simulink model "LinStSpace_org"  (Simulink 10.0)
settings: Solver=ode3  StartTime=0.0  StopTime=20  FixedStep=1  RelTol=1e-3  EnableMultiTasking=on
libraries: Lib_Solve_Linearize_TMATS x1
settings Model: Creator=jwchapm2  LastModifiedBy=annonymous
settings DataIOCC: LimitDataPoints=on  SignalLoggingSaveFormat=ModelDataLogs
settings DebuggingCC: UnderspecifiedInitializationDetection=Simplified  MergeDetectMultiDrivingBlocksExec=error  SolverPrmCheckMsg=warning  MultiTaskDSMMsg=warning  MultiTaskCondExecSysMsg=none  StrictBusMsg=WarnOnBusTreatedAsVector  NonBusSignalsTreatedAsBus=warning
settings GRTTargetCC: GeneratePreprocessorConditionals=Disable all  CombineOutputUpdateFcns=on  GRTInterface=off
settings ConfigComp: CovExternalEMLEnable=off

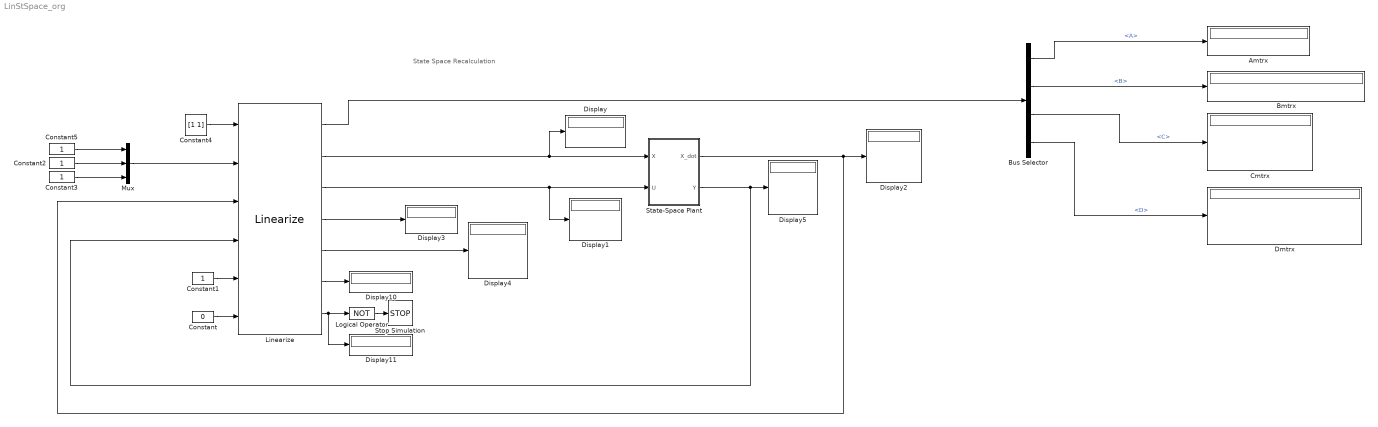
== system LinStSpace_org ==
  note: State Space Recalculation
  Amtrx : Display
  Bmtrx : Display
  Bus Selector : BusSelector  OutputSignals=A,B,C,D
  Cmtrx : Display
  Constant : Constant  Value=0
  Constant{1..3,5} (4 alike) : Constant
  Constant4 : Constant  Value=[1 1]
  Display{,1..5,10..11} (8 alike) : Display
  Dmtrx : Display
  Linearize : Lib_Solve_Linearize_TMATS/Linearize  N_XPer_M=[0.01 0.01;-0.01 -0.01]  N_UPer_M=[0.01 0.01 0.01;-0.01 -0.01 -0.01]  N_Y_M=4
  Logical Operator : Logic  Operator=NOT  AllPortsSameDT=off  OutDataTypeStr=boolean
  Mux : Mux  Inputs=3
  State-Space Plant : Subsystem
  Stop Simulation : Stop
  wires:
  Linearize/2 -> Display/1, State-Space Plant/1(X)
  Linearize/1 -> Bus Selector/1
  Linearize/4 -> Display3/1
  Linearize/5 -> Display4/1
  Constant/1 -> Linearize/6
  Constant4/1 -> Linearize/1
  Constant5/1 -> Mux/1
  Constant2/1 -> Mux/2
  State-Space Plant/2(Y) -> Linearize/4, Display5/1
  State-Space Plant/1(X_dot) -> Linearize/3, Display2/1
  Constant3/1 -> Mux/3
  Bus Selector/1 -> Amtrx/1  "<A>"
  Bus Selector/2 -> Bmtrx/1  "<B>"
  Bus Selector/3 -> Cmtrx/1  "<C>"
  Bus Selector/4 -> Dmtrx/1  "<D>"
  Linearize/6 -> Display10/1
  Linearize/7 -> Display11/1, Logical Operator/1
  Constant1/1 -> Linearize/5
  Mux/1 -> Linearize/2
  Linearize/3 -> Display1/1, State-Space Plant/2("U ")
  Logical Operator/1 -> Stop Simulation/1

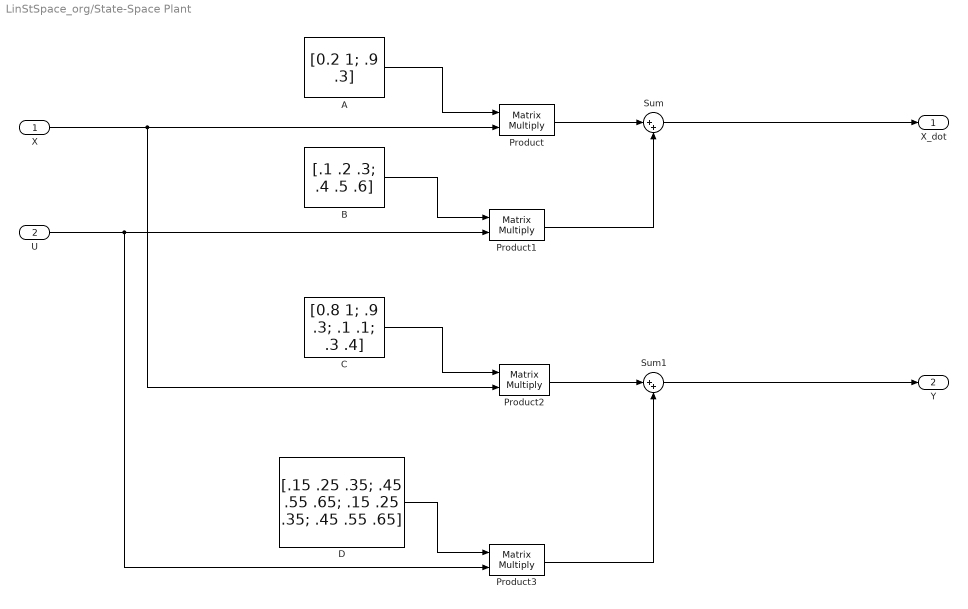
== system LinStSpace_org/State-Space Plant ==
  X : Inport
  "U " : Inport  Port=2
  A : Constant  Value=[0.2 1; .9 .3]
  B : Constant  Value=[.1 .2 .3; .4 .5 .6]
  C : Constant  Value=[0.8 1; .9 .3; .1 .1; .3 .4]
  D : Constant  Value=[.15 .25 .35; .45 .55 .65; .15 .25 .35; .45 .55 .65]
  Product{,1..3} (4 alike) : Product  Multiplication=Matrix(*)
  Sum : Sum  Inputs=|++
  Sum1 : Sum  Inputs=|++
  X_dot : Outport
  Y : Outport  Port=2
  wires:
  Sum/1 -> X_dot/1
  A/1 -> Product/1
  Product/1 -> Sum/1
  B/1 -> Product1/1
  Product1/1 -> Sum/2
  Sum1/1 -> Y/1
  X/1 -> Product2/2, Product/2
  C/1 -> Product2/1
  Product2/1 -> Sum1/1
  D/1 -> Product3/1
  "U "/1 -> Product3/2, Product1/2
  Product3/1 -> Sum1/2
